simulink model "Linear_Frame_Conversion_to_Inertia"  (R2018a)
settings: Solver=VariableStepAuto  StartTime=0.0  StopTime=10.0  RelTol=1e-3
settings Model: Creator=Ibrahim  LastModifiedBy=Ibrahim

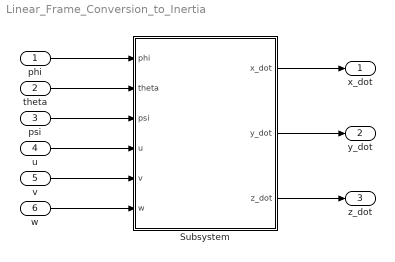
== system Linear_Frame_Conversion_to_Inertia ==
  phi : Inport
  theta : Inport  Port=2
  psi : Inport  Port=3
  u : Inport  Port=4
  v : Inport  Port=5
  w : Inport  Port=6
  Subsystem : Subsystem
  x_dot : Outport
  y_dot : Outport  Port=2
  z_dot : Outport  Port=3
  wires:
  phi/1 -> Subsystem/1(phi)
  theta/1 -> Subsystem/2(theta)
  psi/1 -> Subsystem/3(psi)
  u/1 -> Subsystem/4(u)
  v/1 -> Subsystem/5(v)
  w/1 -> Subsystem/6(w)
  Subsystem/1(x_dot) -> x_dot/1
  Subsystem/2(y_dot) -> y_dot/1
  Subsystem/3(z_dot) -> z_dot/1

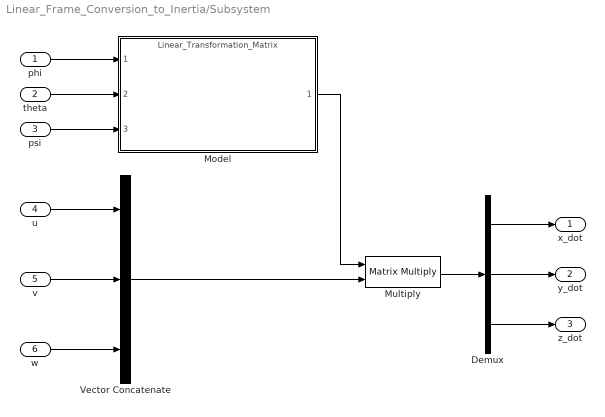
== system Linear_Frame_Conversion_to_Inertia/Subsystem ==
  phi : Inport
  theta : Inport  Port=2
  psi : Inport  Port=3
  u : Inport  Port=4
  v : Inport  Port=5
  w : Inport  Port=6
  Demux : Demux  Outputs=3
  Model : ModelReference  ModelNameDialog=Linear_Transformation_Matrix.slx  SimulationMode=Normal  ModelReferenceVersion=1.3
  Multiply : Product  Multiplication=Matrix(*)
  Vector Concatenate : Concatenate  NumInputs=3
  x_dot : Outport
  y_dot : Outport  Port=2
  z_dot : Outport  Port=3
  wires:
  Model/1 -> Multiply/1
  Vector Concatenate/1 -> Multiply/2
  Multiply/1 -> Demux/1
  Demux/2 -> y_dot/1
  Demux/1 -> x_dot/1
  w/1 -> Vector Concatenate/3
  theta/1 -> Model/2
  v/1 -> Vector Concatenate/2
  psi/1 -> Model/3
  Demux/3 -> z_dot/1
  phi/1 -> Model/1
  u/1 -> Vector Concatenate/1
